simulink model "EinwegGleichrichter_MitFDATool"  (R2014b)
settings: Solver=ode4  StartTime=0.0  StopTime=10  FixedStep=1e-3  MaxStep=1e-4  RelTol=1e-3
libraries: dsparch4 x3
settings Model: Creator=Administrator  LastModifiedBy=Administrator
settings DataIOCC: SignalLoggingSaveFormat=ModelDataLogs  SignalLoggingName=sigsOut
settings DebuggingCC: SaveWithParameterizedLinksMsg=none  UnderspecifiedInitializationDetection=Classic  MergeDetectMultiDrivingBlocksExec=none  SignalResolutionControl=TryResolveAllWithWarning  SolverPrmCheckMsg=none  MultiTaskDSMMsg=warning  MultiTaskCondExecSysMsg=none
settings HardwareCC: TargetUnknown=on
settings RTWCC: IncludeERTFirstTime=on
settings GRTTargetCC: CombineOutputUpdateFcns=off  GRTInterface=on

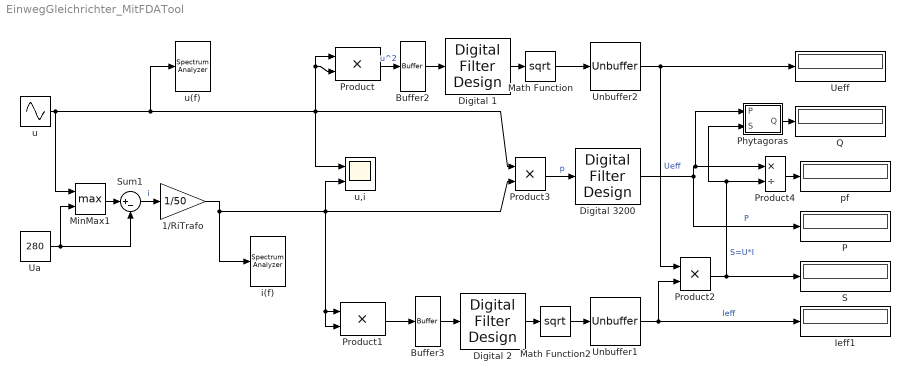
== system EinwegGleichrichter_MitFDATool ==
  1/RiTrafo : Gain  Gain=1/50
  Buffer2 : Buffer  N=256
  Buffer3 : Buffer  N=256
  Digital 1 : dsparch4/Digital Filter Design  mwdsp_browser_bugfix_var=off
  Digital 2 : dsparch4/Digital Filter Design  mwdsp_browser_bugfix_var=off
  Digital 3200 : dsparch4/Digital Filter Design  mwdsp_browser_bugfix_var=off
  Ieff1 : Display
  Math Function : Math  Operator=sqrt  SaturateOnIntegerOverflow=on
  Math Function2 : Math  Operator=sqrt  SaturateOnIntegerOverflow=on
  MinMax1 : MinMax  Function=max  Inputs=2  SaturateOnIntegerOverflow=on  InputSameDT=on
  P : Display
  Phytagoras : Subsystem
  Product{,1..3} (4 alike) : Product  SaturateOnIntegerOverflow=on  OutDataTypeStr=Inherit: Same as first input
  Product4 : Product  Inputs=*/  SaturateOnIntegerOverflow=on  OutDataTypeStr=Inherit: Same as first input
  Q : Display
  S : Display
  Sum1 : Sum  Inputs=|+-  SaturateOnIntegerOverflow=on
  Ua : Constant  Value=280
  Ueff : Display
  Unbuffer1 : Unbuffer
  Unbuffer2 : Unbuffer
  i(f) : SpectrumAnalyzer
  pf : Display
  u : Sin  SineType=Sample based  Amplitude=230*2^0.5  Frequency=314  Samples=20  SampleTime=1e-3
  u(f) : SpectrumAnalyzer
  u,i : Scope  NumInputPorts=2
      settings: YMin=-5~-5  YMax=5~5
  wires:
  Product/1 -> Buffer2/1  "u^2"
  Digital 1/1 -> Math Function/1
  Product1/1 -> Buffer3/1
  Product3/1 -> Digital 3200/1  "p"
  Math Function/1 -> Unbuffer2/1
  u/1 -> Product3/1, Product/2, Product/1, u,i/1, u(f)/1, MinMax1/1
  Buffer2/1 -> Digital 1/1
  Digital 2/1 -> Math Function2/1
  Buffer3/1 -> Digital 2/1
  Math Function2/1 -> Unbuffer1/1
  Unbuffer1/1 -> Ieff1/1, Product2/2  "Ieff"
  Unbuffer2/1 -> Ueff/1, Product2/1  "Ueff"
  Product2/1 -> S/1, Phytagoras/2(S), Product4/2  "S=U*I"
  Product4/1 -> pf/1
  1/RiTrafo/1 -> Product3/2, Product1/1, Product1/2, u,i/2, i(f)/1
  Ua/1 -> MinMax1/2, Sum1/2
  MinMax1/1 -> Sum1/1
  Sum1/1 -> 1/RiTrafo/1  "i"
  Digital 3200/1 -> P/1, Phytagoras/1(P), Product4/1  "P"
  Phytagoras/1(Q) -> Q/1

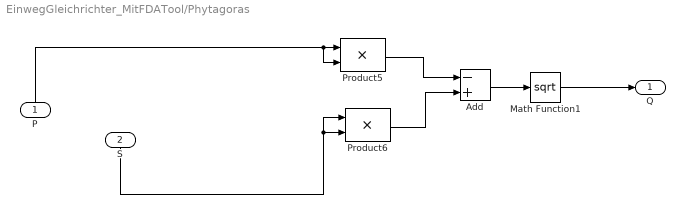
== system EinwegGleichrichter_MitFDATool/Phytagoras ==
  P : Inport
  S : Inport  Port=2
  Add : Sum  Inputs=-+
  Math Function1 : Math  Operator=sqrt  SaturateOnIntegerOverflow=on
  Product5 : Product  SaturateOnIntegerOverflow=on  OutDataTypeStr=Inherit: Same as first input
  Product6 : Product  SaturateOnIntegerOverflow=on  OutDataTypeStr=Inherit: Same as first input
  Q : Outport
  wires:
  Product6/1 -> Add/2
  Product5/1 -> Add/1
  Add/1 -> Math Function1/1
  Math Function1/1 -> Q/1
  P/1 -> Product5/2, Product5/1
  S/1 -> Product6/2, Product6/1
